simulink library "SiPhotonics"  (R2016b)
settings: Solver=ode45  StartTime=0.0  StopTime=10.0  RelTol=1e-3  EnableMultiTasking=on
undefined symbols (not defined in the file): a0, a1, alpha, f0, fref, k_in, L, Lj, n0, n1, Ne, ng, Nh, nt, opt, T0, t_drop, t_in, Vbi, wf
libraries: SiPhotonics x19, powerlib_meascontrol x1
settings Model: Creator=lins08  LastModifiedBy=lins08
settings DataIOCC: LimitDataPoints=on  SaveFormat=Array
settings OptimizationCC: LifeSpan=inf
settings DebuggingCC: SFUnexpectedBacktrackingDiag=warning  SFNoUnconditionalDefaultTransitionDiag=warning  SFExecutionAtInitializationDiag=none
settings HardwareCC: ProdBitPerPointer=32  ProdBitPerSizeT=32  ProdBitPerPtrDiffT=32  ProdLargestAtomicFloat=None  ProdIntDivRoundTo=Undefined  ProdEndianess=Unspecified  ProdWordSize=32  ProdHWDeviceType=32-bit Generic
settings ModelReferenceCC: PropagateSignalLabelsOutOfModel=off
settings GRTTargetCC: TargetLangStandard=C89/C90 (ANSI)  GeneratePreprocessorConditionals=Disable all
settings ConfigComp: CovMetricSettings=dw  CovHtmlReporting=on  CovSaveCumulativeToWorkspaceVar=on  CovSaveSingleToWorkspaceVar=on  CovExternalEMLEnable=off

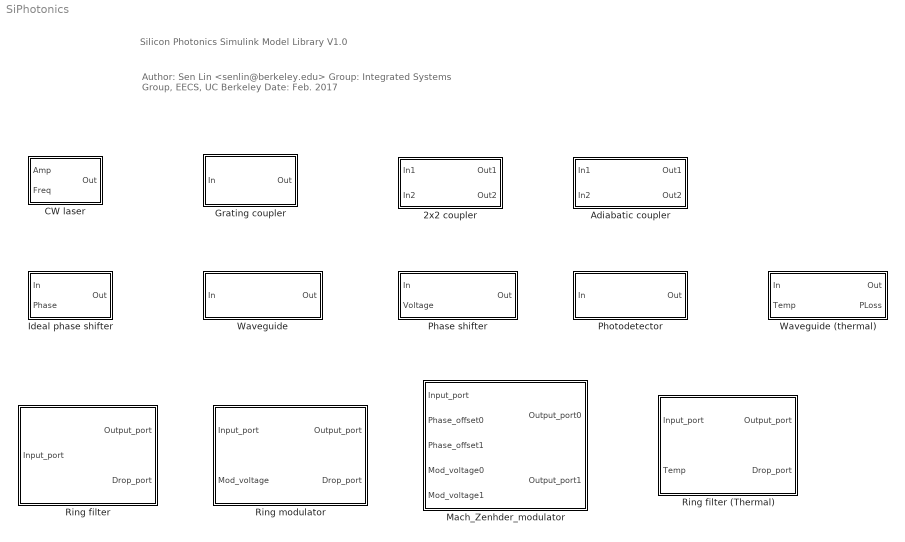
== system SiPhotonics ==
  note: Silicon Photonics Simulink Model Library V1.0
  note: Author: Sen Lin <senlin@berkeley.edu>
      | Group: Integrated Systems Group, EECS, UC Berkeley
      | Date: Feb. 2017
  2x2 coupler : Subsystem  mask{t=t_in, k=k_in}
      mask prompts: t "transmission coef."; k "coupling coef."
  Adiabatic coupler : Subsystem
  CW laser : Subsystem
  Grating coupler : Subsystem  mask{trans=0.3}
      mask prompts: trans "Power Transmission Coef."
  Ideal phase shifter : Subsystem
  Mach_Zenhder_modulator : Subsystem  mask{L=L, fref=fref, n0=n0, ng=ng, n1=n1, a0=a0, a1=a1, Ne=Ne, Nh=Nh, Vbi=Vbi, Lj=Lj, f0=f0, opt=0, wf=0}
      mask prompts: L "Modulation arm (unit: m)"; fref "Reference frequency (Hz)"; n0 "Phase index"; ng "Group index"; n1 "Phase index 1st order (pos)"; a0 "Absorption coef."; a1 "Absorption 1st order (neg)"; Ne "N-doping"; Nh "P-doping"; Vbi "Built-in Voltage"; Lj "Junction geometry factor (cm)"; opt "Model select (1: linear, 2: sqrt, 3: diode)"; wf "waveguide factor"
  Phase shifter : Subsystem  mask{L=1e-6, fref=230e12, n0=2, ng=3, a0=300, c0=3e8, n1=8e-5, a1=-0.3, Ne=5e17, Nh=5e17, Vbi=0.7, Lj=0.5e-4, f0=230e12, opt=opt, wf=wf}
      mask prompts: L "Length of waveguide (unit: m)"; fref "Reference frequency for light"; n0 "Phase index at f0"; ng "Group index"; a0 "Absorption coefficient (/m)"; c0 "Speed of light (m/s)"; n1 "Phase index 1st order (pos)"; a1 "Absorption 1st order (neg)"; Ne "N-doping"; Nh "P-doping"; Vbi "Build-in voltage"; Lj "Junction geometry factor (cm)"; opt "Model (1,2,3)"; wf "Waveguide factor"
      mask DialogControl DescTextVar Prompt: Ideal Phase Shifter
  Photodetector : Subsystem  mask{R=1, fbw=0}
      mask prompts: R "Responsivity Coefficent"; fbw "PD Bandwidth"
  Ring filter : Subsystem  mask{L=L, t_in=t_in, k_in=sqrt(1-t_in^2)*1i, t_drop=t_drop, k_drop=sqrt(1-t_drop^2)*1i, fref=fref, n0=n0, ng=ng, f0=f0, a0=0}
      mask prompts: L "Perimeter (unit: m)"; t_in "Input port transmission coef"; k_in "Input port coupling coef."; t_drop "Drop port transmission coef."; k_drop "Drop port coupling coef."; fref "Reference frequency (Hz)"; n0 "Phase index at f0"; ng "Group index"; a0 "Absorption coeff."
  Ring filter (Thermal) : Subsystem  mask{L=L, t_in=t_in, k_in=sqrt(1-t_in^2)*1i, t_drop=t_drop, k_drop=sqrt(1-t_drop^2)*1i, fref=fref, n0=n0, ng=ng, f0=f0, nt=0, T0=0, gamma_t=0}
      mask prompts: L "Perimeter (unit: m)"; t_in "Input port transmission coef"; k_in "Input port coupling coef."; t_drop "Drop port transmission coef."; k_drop "Drop port coupling coef."; fref "Reference frequency (Hz)"; n0 "Phase index at f0"; ng "Group index"; nt "Thermal coeff."; T0 "Measurement temp"; gamma_t "Power to temp coeff."
  Ring modulator : Subsystem  mask{L=L, t_in=t_in, k_in=sqrt(1-t_in^2)*1i, t_drop=t_drop, k_drop=sqrt(1-t_drop^2)*1i, fref=fref, n0=n0, ng=ng, n1=n1, a0=a0, a1=a1, Ne=Ne, Nh=Nh, Vbi=Vbi, Lj=Lj, f0=f0, opt=opt, wf=0}
      mask prompts: L "Perimeter (unit: m)"; t_in "Input port transmission coef"; k_in "Input port coupling coef."; t_drop "Drop port transmission coef."; k_drop "Drop port coupling coef."; fref "Reference frequency (Hz)"; n0 "Phase index at f0"; ng "Group index"; n1 "Phase index 1st oder (pos)"; a0 "Absorption coefficient (/m)"; a1 "Absorption 1st order (neg)"; Ne "N-doping"; Nh "P-doping"; Vbi "Built-in voltage"; Lj "Junction geometry factor (cm)"; opt "Model (1: linear, 2: sqrt, 3: diode)"; wf "Waveguide factor"
  Waveguide : Subsystem  mask{L=L, fref=fref, n0=n0, ng=ng, a0=alpha, c0=3e8, f0=f0}
      mask prompts: L "Length of waveguide (unit: m)"; fref "Reference frequency for light"; n0 "Phase index at f0"; ng "Group index"; a0 "Absorption coefficient (/cm)"; c0 "Speed of light (m/s)"
      mask DialogControl DescTextVar Prompt: Ideal Phase Shifter
  Waveguide (thermal) : Subsystem  mask{L=L, fref=fref, n0=n0, ng=ng, a0=alpha, c0=3e8, f0=f0, T0=T0, nt=nt}
      mask prompts: L "Length of waveguide (unit: m)"; fref "Reference frequency for light"; n0 "Phase index at f0"; ng "Group index"; a0 "Absorption coefficient (/cm)"; c0 "Speed of light (m/s)"; T0 "Measurement temp (K)"; nt "neff thermal coefficient (/K)"
      mask DialogControl DescTextVar Prompt: Ideal Phase Shifter

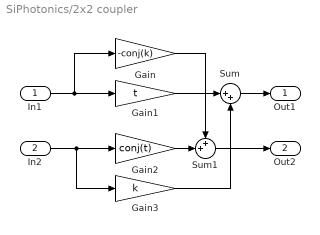
== system SiPhotonics/2x2 coupler ==
  In1 : Inport
      settings: SignalType=complex
  In2 : Inport  Port=2
      settings: SignalType=complex
  Gain : Gain  Gain=-conj(k)
  Gain1 : Gain  Gain=t
  Gain2 : Gain  Gain=conj(t)
  Gain3 : Gain  Gain=k
  Sum : Sum  Inputs=|++
  Sum1 : Sum  Inputs=++|
  Out1 : Outport
      settings: SignalType=complex
  Out2 : Outport  Port=2
      settings: SignalType=complex
  wires:
  In1/1 -> Gain/1, Gain1/1
  In2/1 -> Gain3/1, Gain2/1
  Gain1/1 -> Sum/1
  Sum/1 -> Out1/1
  Gain3/1 -> Sum/2
  Gain2/1 -> Sum1/2
  Sum1/1 -> Out2/1
  Gain/1 -> Sum1/1

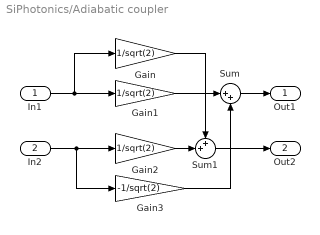
== system SiPhotonics/Adiabatic coupler ==
  In1 : Inport
      settings: SignalType=complex
  In2 : Inport  Port=2
      settings: SignalType=complex
  Gain : Gain  Gain=1/sqrt(2)
  Gain1 : Gain  Gain=1/sqrt(2)
  Gain2 : Gain  Gain=1/sqrt(2)
  Gain3 : Gain  Gain=-1/sqrt(2)
  Sum : Sum  Inputs=|++
  Sum1 : Sum  Inputs=++|
  Out1 : Outport
      settings: SignalType=complex
  Out2 : Outport  Port=2
      settings: SignalType=complex
  wires:
  In1/1 -> Gain/1, Gain1/1
  In2/1 -> Gain3/1, Gain2/1
  Gain1/1 -> Sum/1
  Sum/1 -> Out1/1
  Gain3/1 -> Sum/2
  Gain2/1 -> Sum1/2
  Sum1/1 -> Out2/1
  Gain/1 -> Sum1/1

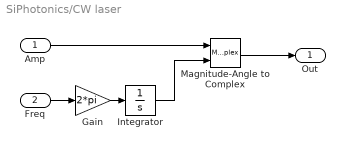
== system SiPhotonics/CW laser ==
  Amp : Inport
  Freq : Inport  Port=2
  Gain : Gain  Gain=2*pi
  Integrator : Integrator
  Magnitude-Angle to Complex : MagnitudeAngleToComplex
  Out : Outport
      settings: SignalType=complex
  wires:
  Magnitude-Angle to Complex/1 -> Out/1
  Integrator/1 -> Magnitude-Angle to Complex/2
  Gain/1 -> Integrator/1
  Freq/1 -> Gain/1
  Amp/1 -> Magnitude-Angle to Complex/1

== system SiPhotonics/Grating coupler ==
  In : Inport
  Gain : Gain  Gain=sqrt(trans)
  Out : Outport
  wires:
  In/1 -> Gain/1
  Gain/1 -> Out/1

== system SiPhotonics/Ideal phase shifter ==
  In : Inport
      settings: SignalType=complex
  Phase : Inport  Port=2
  Complex to Magnitude-Angle : ComplexToMagnitudeAngle
  Magnitude-Angle to Complex : MagnitudeAngleToComplex
  Sum : Sum  Inputs=|++
  Out : Outport
      settings: SignalType=complex
  wires:
  In/1 -> Complex to Magnitude-Angle/1
  Complex to Magnitude-Angle/2 -> Sum/1
  Complex to Magnitude-Angle/1 -> Magnitude-Angle to Complex/1
  Magnitude-Angle to Complex/1 -> Out/1
  Sum/1 -> Magnitude-Angle to Complex/2
  Phase/1 -> Sum/2

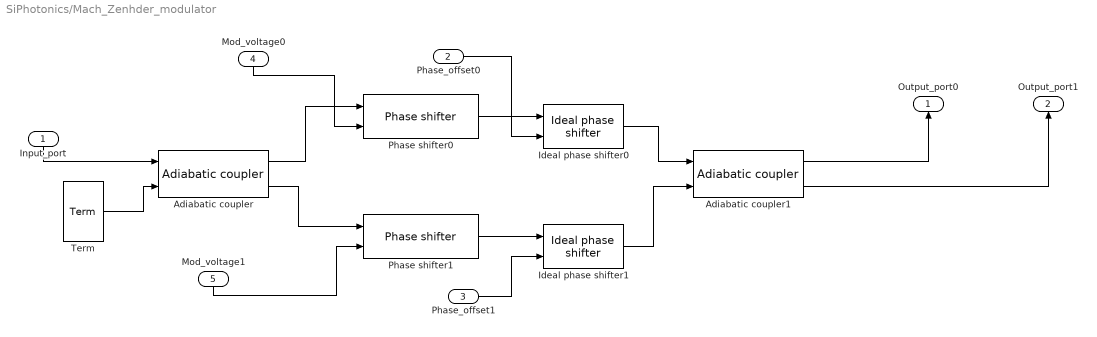
== system SiPhotonics/Mach_Zenhder_modulator ==
  Input_port : Inport
  Phase_offset0 : Inport  Port=2
  Phase_offset1 : Inport  Port=3
  Mod_voltage0 : Inport  Port=4
  Mod_voltage1 : Inport  Port=5
  Adiabatic coupler : SiPhotonics/Adiabatic coupler
  Adiabatic coupler1 : SiPhotonics/Adiabatic coupler
  Ideal phase shifter0 : SiPhotonics/Ideal phase shifter
  Ideal phase shifter1 : SiPhotonics/Ideal phase shifter
  Phase shifter0 : SiPhotonics/Phase shifter  L=L  fref=fref  n0=n0  ng=ng  a0=a0  c0=3e8  n1=n1  a1=a1  Ne=Ne  Nh=Nh  Vbi=Vbi  Lj=Lj  f0=f0  opt=opt
  Phase shifter1 : SiPhotonics/Phase shifter  L=L  fref=fref  n0=n0  ng=ng  a0=a0  c0=3e8  n1=n1  a1=a1  Ne=Ne  Nh=Nh  Vbi=Vbi  Lj=Lj  f0=f0  opt=opt
  Term : SiPhotonics/Ring modulator/Term
  Output_port0 : Outport
  Output_port1 : Outport  Port=2
  wires:
  Input_port/1 -> Adiabatic coupler/1
  Mod_voltage1/1 -> Phase shifter1/2
  Term/1 -> Adiabatic coupler/2
  Adiabatic coupler1/2 -> Output_port1/1
  Adiabatic coupler/1 -> Phase shifter0/1
  Adiabatic coupler/2 -> Phase shifter1/1
  Mod_voltage0/1 -> Phase shifter0/2
  Phase shifter1/1 -> Ideal phase shifter1/1
  Ideal phase shifter1/1 -> Adiabatic coupler1/2
  Adiabatic coupler1/1 -> Output_port0/1
  Phase_offset1/1 -> Ideal phase shifter1/2
  Phase shifter0/1 -> Ideal phase shifter0/1
  Ideal phase shifter0/1 -> Adiabatic coupler1/1
  Phase_offset0/1 -> Ideal phase shifter0/2

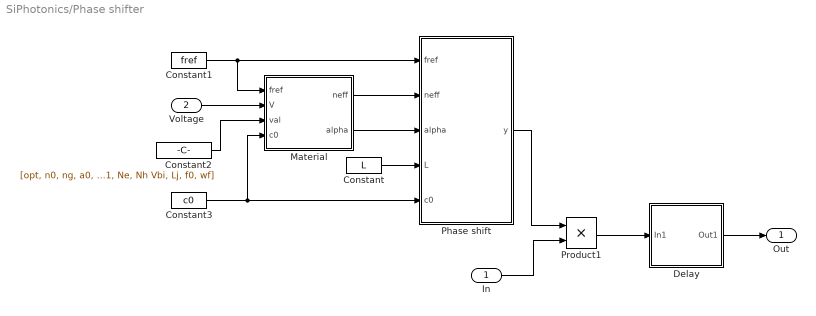
== system SiPhotonics/Phase shifter ==
  In : Inport
      settings: SignalType=complex
  Voltage : Inport  Port=2
  Constant : Constant  Value=L
  Constant1 : Constant  Value=fref
  Constant2 : Constant  Value=[opt, n0, ng, a0, n1, a1, Ne, Nh Vbi, Lj, f0, wf]
  Constant3 : Constant  Value=c0
  Delay : Subsystem
  Material : MATLAB Function  TreatAsAtomicUnit=on
  Phase shift : MATLAB Function  TreatAsAtomicUnit=on
  Product1 : Product
  Out : Outport
      settings: SignalType=complex
  wires:
  In/1 -> Product1/2
  Phase shift/1(y) -> Product1/1
  Constant/1 -> Phase shift/4(L)
  Constant1/1 -> Material/1(fref), Phase shift/1(fref)
  Constant3/1 -> Material/4(c0), Phase shift/5(c0)
  Product1/1 -> Delay/1(In1)
  Delay/1(Out1) -> Out/1
  Material/1(neff) -> Phase shift/2(neff)
  Material/2(alpha) -> Phase shift/3(alpha)
  Voltage/1 -> Material/2(V)
  Constant2/1 -> Material/3(val)

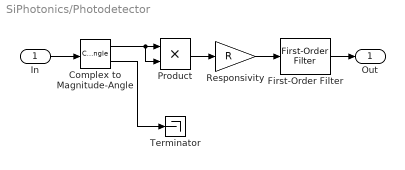
== system SiPhotonics/Photodetector ==
  In : Inport
  Complex to Magnitude-Angle : ComplexToMagnitudeAngle
  First-Order Filter : powerlib_meascontrol/Filters/First-Order Filter  FilterType=Lowpass  Tc=1/(2*pi*fbw)  Ts=0  Initialize=on  Vac_Init=[0, 0, 60]  Vdc_Init=0  PlotResponse=off  FreqRange="[0,  200,  1]"
  Product : Product
  Responsivity : Gain  Gain=R
  Terminator : Terminator
  Out : Outport
  wires:
  In/1 -> Complex to Magnitude-Angle/1
  Complex to Magnitude-Angle/1 -> Product/2, Product/1
  Product/1 -> Responsivity/1
  Responsivity/1 -> First-Order Filter/1
  First-Order Filter/1 -> Out/1
  Complex to Magnitude-Angle/2 -> Terminator/1

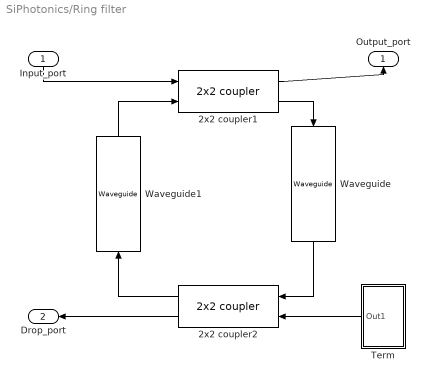
== system SiPhotonics/Ring filter ==
  Input_port : Inport
  2x2 coupler1 : SiPhotonics/2x2 coupler  t=t_in  k=k_in
  2x2 coupler2 : SiPhotonics/2x2 coupler  t=t_drop  k=k_drop
  Term : Subsystem
  Waveguide : SiPhotonics/Waveguide  L=L/2  fref=fref  n0=n0  ng=ng  a0=a0  c0=3e8  f0=f0
  Waveguide1 : SiPhotonics/Waveguide  L=L/2  fref=fref  n0=n0  ng=ng  a0=a0  c0=3e8  f0=f0
  Output_port : Outport
  Drop_port : Outport  Port=2
  wires:
  Waveguide1/1 -> 2x2 coupler1/2
  2x2 coupler2/1 -> Waveguide1/1
  Input_port/1 -> 2x2 coupler1/1
  2x2 coupler2/2 -> Drop_port/1
  2x2 coupler1/2 -> Waveguide/1
  2x2 coupler1/1 -> Output_port/1
  Waveguide/1 -> 2x2 coupler2/1
  Term/1(Out1) -> 2x2 coupler2/2

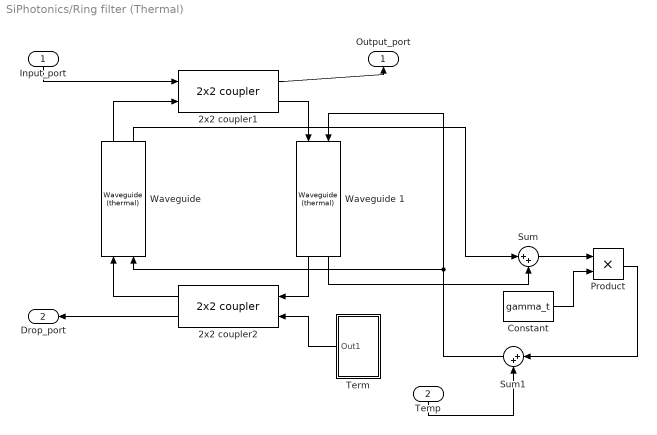
== system SiPhotonics/Ring filter (Thermal) ==
  Input_port : Inport
  Temp : Inport  Port=2
  2x2 coupler1 : SiPhotonics/2x2 coupler  t=t_in  k=k_in
  2x2 coupler2 : SiPhotonics/2x2 coupler  t=t_drop  k=k_drop
  Constant : Constant  Value=gamma_t
  Product : Product
  Sum : Sum  Inputs=|++
  Sum1 : Sum  Inputs=|++
  Term : Subsystem
  Waveguide : SiPhotonics/Waveguide (thermal)  L=L/2  fref=fref  n0=n0  ng=ng  a0=a0  c0=3e8  f0=f0  T0=T0  nt=nt
  Waveguide 1 : SiPhotonics/Waveguide (thermal)  L=L/2  fref=fref  n0=n0  ng=ng  a0=a0  c0=3e8  f0=f0  T0=T0  nt=nt
  Output_port : Outport
  Drop_port : Outport  Port=2
  wires:
  Term/1(Out1) -> 2x2 coupler2/2
  Waveguide 1/1 -> 2x2 coupler2/1
  2x2 coupler1/1 -> Output_port/1
  2x2 coupler1/2 -> Waveguide 1/1
  2x2 coupler2/2 -> Drop_port/1
  Input_port/1 -> 2x2 coupler1/1
  2x2 coupler2/1 -> Waveguide/1
  Waveguide/1 -> 2x2 coupler1/2
  Waveguide/2 -> Sum/1
  Waveguide 1/2 -> Sum/2
  Sum/1 -> Product/1
  Constant/1 -> Product/2
  Product/1 -> Sum1/1
  Sum1/1 -> Waveguide/2, Waveguide 1/2
  Temp/1 -> Sum1/2

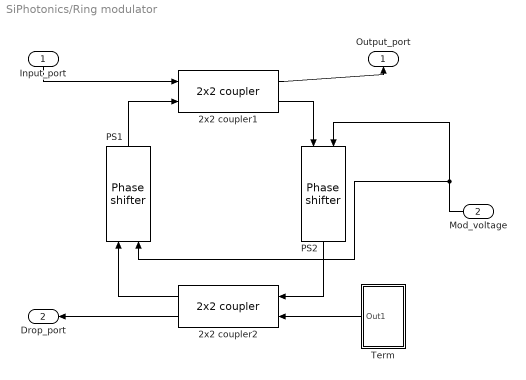
== system SiPhotonics/Ring modulator ==
  Input_port : Inport
  Mod_voltage : Inport  Port=2
  2x2 coupler1 : SiPhotonics/2x2 coupler  t=t_in  k=k_in
  2x2 coupler2 : SiPhotonics/2x2 coupler  t=t_drop  k=k_drop
  PS1 : SiPhotonics/Phase shifter  L=L/2  fref=fref  n0=n0  ng=ng  a0=a0  c0=3e8  n1=n1  a1=a1  Ne=Ne  Nh=Nh  Vbi=Vbi  Lj=Lj  f0=f0  opt=opt  wf=wf
  PS2 : SiPhotonics/Phase shifter  L=L/2  fref=fref  n0=n0  ng=ng  a0=a0  c0=3e8  n1=n1  a1=a1  Ne=Ne  Nh=Nh  Vbi=Vbi  Lj=Lj  f0=f0  opt=opt  wf=wf
  Term : Subsystem
  Output_port : Outport
  Drop_port : Outport  Port=2
  wires:
  PS1/1 -> 2x2 coupler1/2
  2x2 coupler2/1 -> PS1/1
  Input_port/1 -> 2x2 coupler1/1
  2x2 coupler2/2 -> Drop_port/1
  2x2 coupler1/2 -> PS2/1
  2x2 coupler1/1 -> Output_port/1
  PS2/1 -> 2x2 coupler2/1
  Term/1(Out1) -> 2x2 coupler2/2
  Mod_voltage/1 -> PS1/2, PS2/2

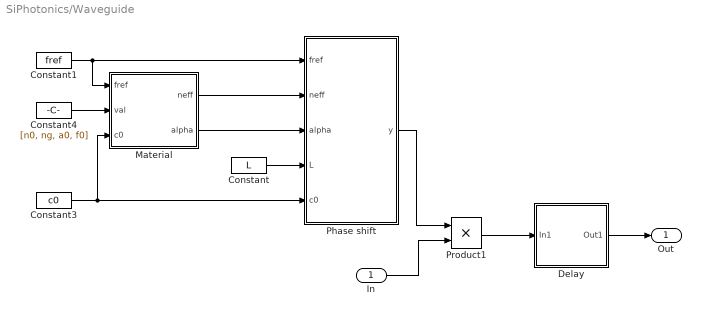
== system SiPhotonics/Waveguide ==
  In : Inport
      settings: SignalType=complex
  Constant : Constant  Value=L
  Constant1 : Constant  Value=fref
  Constant3 : Constant  Value=c0
  Constant4 : Constant  Value=[n0, ng, a0, f0]
  Delay : Subsystem
  Material : MATLAB Function  TreatAsAtomicUnit=on
  Phase shift : MATLAB Function  TreatAsAtomicUnit=on
  Product1 : Product
  Out : Outport
      settings: SignalType=complex
  wires:
  Material/2(alpha) -> Phase shift/3(alpha)
  Material/1(neff) -> Phase shift/2(neff)
  Delay/1(Out1) -> Out/1
  Product1/1 -> Delay/1(In1)
  Constant3/1 -> Material/3(c0), Phase shift/5(c0)
  Constant1/1 -> Material/1(fref), Phase shift/1(fref)
  Constant/1 -> Phase shift/4(L)
  Phase shift/1(y) -> Product1/1
  In/1 -> Product1/2
  Constant4/1 -> Material/2(val)

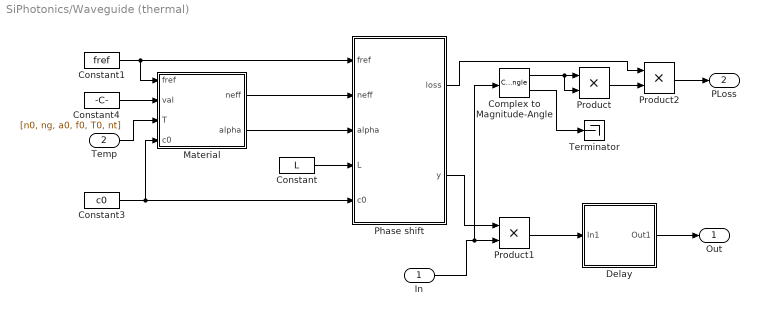
== system SiPhotonics/Waveguide (thermal) ==
  In : Inport
      settings: SignalType=complex
  Temp : Inport  Port=2
  Complex to Magnitude-Angle : ComplexToMagnitudeAngle
  Constant : Constant  Value=L
  Constant1 : Constant  Value=fref
  Constant3 : Constant  Value=c0
  Constant4 : Constant  Value=[n0, ng, a0, f0, T0, nt]
  Delay : Subsystem
  Material : MATLAB Function  TreatAsAtomicUnit=on
  Phase shift : MATLAB Function  TreatAsAtomicUnit=on
  Product : Product
  Product1 : Product
  Product2 : Product
  Terminator : Terminator
  Out : Outport
      settings: SignalType=complex
  PLoss : Outport  Port=2
  wires:
  Material/2(alpha) -> Phase shift/3(alpha)
  Material/1(neff) -> Phase shift/2(neff)
  Delay/1(Out1) -> Out/1
  Product1/1 -> Delay/1(In1)
  Constant3/1 -> Material/4(c0), Phase shift/5(c0)
  Constant1/1 -> Material/1(fref), Phase shift/1(fref)
  Constant/1 -> Phase shift/4(L)
  Phase shift/2(y) -> Product1/1
  Constant4/1 -> Material/2(val)
  Temp/1 -> Material/3(T)
  In/1 -> Complex to Magnitude-Angle/1, Product1/2
  Complex to Magnitude-Angle/1 -> Product/2, Product/1
  Product/1 -> Product2/2
  Complex to Magnitude-Angle/2 -> Terminator/1
  Phase shift/1(loss) -> Product2/1
  Product2/1 -> PLoss/1

== system SiPhotonics/Phase shifter/Delay ==
  In1 : Inport
  Complex to Real-Imag1 : ComplexToRealImag
  Real-Imag to Complex1 : RealImagToComplex
  Transport Delay : TransportDelay  DelayTime=L*ng/c0
  Transport Delay1 : TransportDelay  DelayTime=L*ng/c0
  Out1 : Outport
  wires:
  Real-Imag to Complex1/1 -> Out1/1
  Transport Delay1/1 -> Real-Imag to Complex1/2
  Complex to Real-Imag1/1 -> Transport Delay/1
  In1/1 -> Complex to Real-Imag1/1
  Complex to Real-Imag1/2 -> Transport Delay1/1
  Transport Delay/1 -> Real-Imag to Complex1/1

== system SiPhotonics/Ring filter/Term ==
  Constant : Constant  Value=0
  Constant1 : Constant  Value=0
  Real-Imag to Complex : RealImagToComplex
  Out1 : Outport
  wires:
  Constant/1 -> Real-Imag to Complex/1
  Constant1/1 -> Real-Imag to Complex/2
  Real-Imag to Complex/1 -> Out1/1

== system SiPhotonics/Ring filter (Thermal)/Term ==
  Constant : Constant  Value=0
  Constant1 : Constant  Value=0
  Real-Imag to Complex : RealImagToComplex
  Out1 : Outport
  wires:
  Real-Imag to Complex/1 -> Out1/1
  Constant1/1 -> Real-Imag to Complex/2
  Constant/1 -> Real-Imag to Complex/1

== system SiPhotonics/Ring modulator/Term ==
  Constant : Constant  Value=0
  Constant1 : Constant  Value=0
  Real-Imag to Complex : RealImagToComplex
  Out1 : Outport
  wires:
  Constant/1 -> Real-Imag to Complex/1
  Constant1/1 -> Real-Imag to Complex/2
  Real-Imag to Complex/1 -> Out1/1

== system SiPhotonics/Waveguide/Delay ==
  In1 : Inport
  Complex to Real-Imag1 : ComplexToRealImag
  Real-Imag to Complex1 : RealImagToComplex
  Transport Delay : TransportDelay  DelayTime=L*ng/c0
  Transport Delay1 : TransportDelay  DelayTime=L*ng/c0
  Out1 : Outport
  wires:
  Transport Delay/1 -> Real-Imag to Complex1/1
  Complex to Real-Imag1/2 -> Transport Delay1/1
  In1/1 -> Complex to Real-Imag1/1
  Complex to Real-Imag1/1 -> Transport Delay/1
  Transport Delay1/1 -> Real-Imag to Complex1/2
  Real-Imag to Complex1/1 -> Out1/1

== system SiPhotonics/Waveguide (thermal)/Delay ==
  In1 : Inport
  Complex to Real-Imag1 : ComplexToRealImag
  Real-Imag to Complex1 : RealImagToComplex
  Transport Delay : TransportDelay  DelayTime=L*ng/c0
  Transport Delay1 : TransportDelay  DelayTime=L*ng/c0
  Out1 : Outport
  wires:
  Transport Delay/1 -> Real-Imag to Complex1/1
  Complex to Real-Imag1/2 -> Transport Delay1/1
  In1/1 -> Complex to Real-Imag1/1
  Complex to Real-Imag1/1 -> Transport Delay/1
  Transport Delay1/1 -> Real-Imag to Complex1/2
  Real-Imag to Complex1/1 -> Out1/1

== matlab function SiPhotonics/Phase shifter/Material ==
  data: fref input; V input; neff output; val input; alpha output; c0 input
function [neff, alpha] = fmat(fref, V, val, c0)

model_select = val(1); 
% model selection
% 1--linear, 2--sqrt, 3--diode
n0 = val(2);  % effective refractive index measured at f0
ng = val(3);  % group index
a0 = val(4);  % absorption coefficient in m^-1
n1 = val(5);  % positive
a1 = val(6);  % negative
Nd = val(7);  % n-doping
Na = val(8);  % p-doping
Vbi = val(9); % build-in voltage
Lj = val(10); % geometry/mode factor (cm)
f0 = val(11); % measurement frequency
wf = val(12);  % waveguide factor

% define constants
eps = 11.68*8.85e-14;  % silicon permitivity F/cm
q = 1.602e-19;         % electron charge      
lam0 = c0/f0;

% update refractive index at fref
dlam = (c0/fref-c0/f0);
n0 = n0 + dlam*(n0-ng)/lam0;

% Soref & Bennett, 1987, unit: cm
A = lam0^2*3.64e-10;
B = lam0^2*3.51e-6;
C = 1/2*lam0^2*3.52e-6;  
D = 1/2*lam0^2*2.4e-6;
% 1/2 factor converting power coef. to field coef.


switch model_select
    case 1
        neff = n0 + n1*(-V);
        alpha = a0 + a1*(-V);
        
    case 2
        neff = n0 + n1*sqrt(Vbi-V);
        alpha = a0 + a1*sqrt(Vbi-V);
        
    case 3
        Vbi = 0.0259*log(Nd*Na/10^20);
        xp = sqrt(2*eps*Nd/(q*Na*(Nd+Na))*(Vbi-V));
        xn = sqrt(2*eps*Na/(q*Nd*(Nd+Na))*(Vbi-V));    
        % update n0, a0
        n0 = n0 - (A*Nd + B*Na^0.8)/2 * wf;
        a0 = a0 + 100*(C*Nd + D*Na)/2 * wf;
        neff = n0 + (xp*B*Na^0.8 + xn*A*Nd)/Lj * wf;
        alpha = a0 - 100*(xp*D*Na + xn*C*Nd)/Lj * wf;
        
    otherwise
        neff = n0;
        alpha = a0;
end
%#codegen

== matlab function SiPhotonics/Waveguide/Material ==
  data: fref input; neff output; val input; c0 input; alpha output
function [neff, alpha] = fmat(fref, val, c0)

n0 = val(1);  % effective refractive index measured at f0
ng = val(2);  % group index
a0 = val(3);
f0 = val(4); % measurement frequency    
lam0 = c0/f0;
% update refractive index at fref
dlam = (c0/fref-c0/f0);
neff = n0 + dlam*(n0-ng)/lam0;
alpha = a0;

end
%#codegen

== matlab function SiPhotonics/Waveguide/Phase shift ==
  data: fref input; neff input; alpha input; y output; L input; c0 input
function y = fp(fref, neff, alpha, L, c0)
%#codegen
y = exp(-1i*(L*neff*2*pi*fref/c0)-alpha*L);

== matlab function SiPhotonics/Phase shifter/Phase shift ==
  data: fref input; neff input; alpha input; y output; L input; c0 input
function y = fp(fref, neff, alpha, L, c0)
%#codegen
y = exp(-1i*(L*neff*2*pi*fref/c0)-alpha*L);

== matlab function SiPhotonics/Waveguide (thermal)/Material ==
  data: fref input; neff output; val input; T input; c0 input; alpha output
function [neff, alpha] = fmat(fref, val, T, c0)

n0 = val(1); % effective refractive index measured at f0
ng = val(2); % group index
a0 = val(3);
f0 = val(4); % measurement frequency
T0 = val(5); % measurement temperature, usually room temperature
nt = val(6); % time-dependence of refractive index
lam0 = c0/f0;
% update refractive index at fref
dlam = (c0/fref-c0/f0);
neff = n0 + dlam*(n0-ng)/lam0 + (T-T0)*nt;
alpha = a0;

end
%#codegen

== matlab function SiPhotonics/Waveguide (thermal)/Phase shift ==
  data: loss output; fref input; neff input; alpha input; y output; L input; c0 input
function [loss, y] = fp(fref, neff, alpha, L, c0)
%#codegen
y = exp(-1i*(L*neff*2*pi*fref/c0)-alpha*L);
loss = 1-exp(-2*alpha*L);
